simulink model "PWM"  (R2020b)
settings: Solver=VariableStepAuto  StartTime=0.0  StopTime=0.06  RelTol=1e-3
libraries: powerlib x11, simulink x2, powerlib_meascontrol x1
settings Model: Creator=Anuj Attri  LastModifiedBy=Anuj Attri

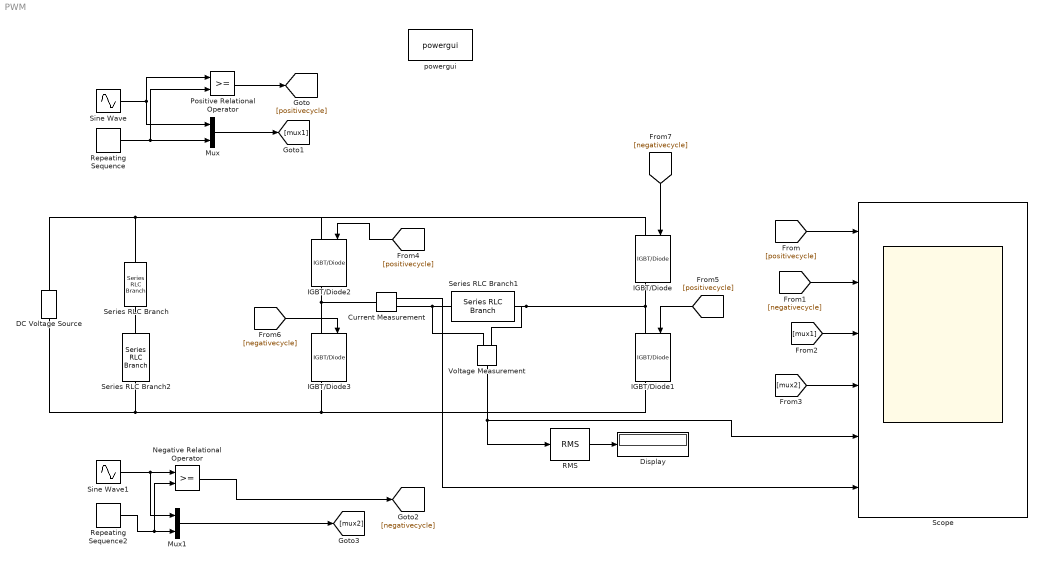
== system PWM ==
  Current Measurement : powerlib/Measurements/Current Measurement  PhasorSimulation=off  OutputType=Complex  PSBequivalent=0
  DC Voltage Source : powerlib/Electrical Sources/DC Voltage Source  Amplitude=230  Measurements=Voltage
  Display : Display
  IGBT/Diode{,1..3} (4 alike) : powerlib/Power Electronics/IGBT//Diode  Ron=1e-3  Rs=1e5  Cs=inf  Measurements=on
  Mux : Mux  Inputs=2
  Mux1 : Mux  Inputs=2
  Negative Relational Operator : RelationalOperator  OutDataTypeStr=boolean  ZeroCross=off  RndMeth=Simplest
  Positive Relational Operator : RelationalOperator  OutDataTypeStr=boolean  ZeroCross=off  RndMeth=Simplest
  RMS : powerlib_meascontrol/Measurements/RMS  TrueRMS=on  Freq=50  RMSInit=0  Ts=0
  Repeating Sequence : simulink/Sources/Repeating Sequence  rep_seq_t=[0, 0.1e-3, 0.2e-3]  rep_seq_y=[0 1 0]
  Repeating Sequence2 : simulink/Sources/Repeating Sequence  rep_seq_t=[0, 0.1e-3, 0.2e-3]  rep_seq_y=[0 1 0]
  Scope : Scope  NumInputPorts=6
  Series RLC Branch : powerlib/Elements/Series RLC Branch  LConnTagsString=__new0  RConnTagsString=__new0  BranchType=C  Resistance=0.1  Inductance=1e-3  SetiL0=off  InitialCurrent=0  Capacitance=100e-6  Setx0=on  InitialVoltage=0  Measurements=None
  Series RLC Branch1 : powerlib/Elements/Series RLC Branch  LConnTagsString=__new0  RConnTagsString=__new0  BranchType=R  Resistance=100  Inductance=1e-3  SetiL0=off  InitialCurrent=0  Capacitance=100e-6  Setx0=off  InitialVoltage=0  Measurements=None
  Series RLC Branch2 : powerlib/Elements/Series RLC Branch  LConnTagsString=__new0  RConnTagsString=__new0  BranchType=R  Resistance=0.1  Inductance=1e-3  SetiL0=off  InitialCurrent=0  Capacitance=100e-6  Setx0=off  InitialVoltage=0  Measurements=None
  Sine Wave : Sin  Amplitude=0.8  Frequency=314  SampleTime=2e-6
  Sine Wave1 : Sin  Amplitude=-0.8  Frequency=314  SampleTime=2e-6
  Voltage Measurement : powerlib/Measurements/Voltage Measurement  PhasorSimulation=off  OutputType=Complex  PSBequivalent=0
  powergui : powerlib/powergui  Priority=1  SimulationMode=Continuous  SampleTime=50e-6  frequency=60  Iterations=50  frequencyindice=0  Pbase=100e6  ErrMax=1e-4  UnitsV=kV  UnitsW=MW  buscounter=0  FunctionMessages=off  echomessages=off  EnableUseOfTLC=off  CurrentSourceSwitches=off  DisableSnubberDevices=on  DisableRonSwitches=off  DisableVfSwitches=off  DisplayEquations=off  AutomaticDiscreteSolvers=off  SolverType=Tustin/Backward Euler (TBE)  Interpol=off  ExternalGateDelay=off  methode=off  Ts=100  x0status=blocks  SPID=on  SwTol=0  HookPort=off  NonlinearTolerance=1e-4  nMaxIteration=100  ContinueOnMaxIteration=off  RestoreLinks=warning  ResistiveCurrentMeasurement=off  Frange=[0:2:500]  Ylog=off  Xlog=on  ShowGrid=off  save=off  variable=ZData  structure=0  ZoomFFT=off  StartTime=0.0  cycles=1  DisplayStyle=1  fundamental=60  FreqAxis=off  MaxFrequency=1000  frequencyindicesteady=1  RmsSteady=1  display=off
  wires:
  Sine Wave/1 -> Positive Relational Operator/1, Mux/1
  Repeating Sequence/1 -> Positive Relational Operator/2, Mux/2
  Sine Wave1/1 -> Negative Relational Operator/1, Mux1/1
  Repeating Sequence2/1 -> Negative Relational Operator/2, Mux1/2
  RMS/1 -> Display/1
  Voltage Measurement/1 -> Scope/5, RMS/1
  Current Measurement/1 -> Scope/6
  Negative Relational Operator/1 -> [negativecycle]
  Positive Relational Operator/1 -> [positivecycle]
  Mux/1 -> [mux1]
  [positivecycle] -> IGBT/Diode1/1
  [positivecycle] -> IGBT/Diode2/1
  Mux1/1 -> [mux2]
  [mux2] -> Scope/4
  [mux1] -> Scope/3
  [negativecycle] -> Scope/2
  [positivecycle] -> Scope/1
  [negativecycle] -> IGBT/Diode/1
  [negativecycle] -> IGBT/Diode3/1
  connections:
  IGBT/Diode2/LConn1 -- IGBT/Diode/LConn1 -- Series RLC Branch/LConn1 -- DC Voltage Source/RConn1
  Series RLC Branch1/LConn1 -- Voltage Measurement/LConn1 -- IGBT/Diode1/LConn1 -- IGBT/Diode/RConn1
  DC Voltage Source/LConn1 -- IGBT/Diode1/RConn1 -- IGBT/Diode3/RConn1 -- Series RLC Branch2/LConn1
  Current Measurement/LConn1 -- IGBT/Diode3/LConn1 -- IGBT/Diode2/RConn1
  Current Measurement/RConn1 -- Voltage Measurement/LConn2 -- Series RLC Branch1/RConn1
  Series RLC Branch/RConn1 -- Series RLC Branch2/RConn1
